simulink model "CtrlCmdCalc"  (R2022b)
settings: Solver=FixedStepDiscrete  StartTime=0.0  StopTime=10.0  FixedStep=0.0001  RelTol=1e-3
values from neighbouring files (symbols this model uses):
  Trq_coeff_Arr_Back_60V = 0.0    [MCU_CtrlCmd.sldd]    (also in MCU_CtrlCmd_objects.m = myPackage.Parameter)
  Trq_coeff_Arr_Back_72V = 0.0    [MCU_CtrlCmd.sldd]    (also in MCU_CtrlCmd_objects.m = myPackage.Parameter)
  Trq_coeff_Arr_HSP_60V = 0.0    [MCU_CtrlCmd.sldd]    (also in MCU_CtrlCmd_objects.m = myPackage.Parameter)
  Trq_coeff_Arr_HSP_72V = 0.0    [MCU_CtrlCmd.sldd]    (also in MCU_CtrlCmd_objects.m = myPackage.Parameter)
  TWISTGRIP_HIGH = 3.3    [MCU_CtrlCmd.sldd]
undefined symbols (not defined in the file or in its folder): ANALOG, cNoneMode, cSpeedLoopMode, cTorqueLoopMode, GEAR, MOTORDIR, ParamCfg_CommandSource_u16, ParamCfg_MaxTorque_u16, POWER_ON, PTIME, STANDBY, TWISTGRIP_UP, TWISTGRIP_VTH_HIGH, TWISTGRIP_VTH_UP
libraries: simulink x2
(part 2 of 2)

== stateflow chart CtrlCmdCalc/CtrlCmd/AntiTheft_HDC/Calc/Chart ==
  (default) -> (junction 5)
  (junction 5) -> (junction 7) [order 1] : [AntiTheftFlag==true]
  (junction 5) -> (junction 9) [order 2]
  (junction 7) -> (junction 9) : {
      | ModeCmd =cSpeedLoopMode;
      | SpeedCmd = 0;
      | RunCmd = 1
      | }
  (junction 9) -> (junction 16)
  (junction 16) -> (junction 18) [order 1] : [HDCState==0 && TGFlag==false && BrakeState==false]
  (junction 16) -> (junction 26) [order 2]
  (junction 18) -> (junction 23) : {
      | ModeCmd=cSpeedLoopMode;
      | RunCmd = 1
      | }
  (junction 23) -> (junction 20) [order 2] : {SpeedCmd=-1200}
  (junction 23) -> (junction 20) [order 1] : [MOTORDIR]{SpeedCmd=1200}
  (junction 20) -> (junction 26)
  (junction 26) -> (junction 28)
  data: AntiTheftFlag input; HDCState input; TGFlag input; BrakeState input; ModeCmd output uint16 =0; cSpeedLoopMode parameter; RunCmd output uint16; SpeedCmd output single; MOTORDIR parameter
